simulink model "Fixed_Wing_Model"  (R2023a)
settings: Solver=FixedStepAuto  StartTime=0.0  StopTime=inf  FixedStep=model_sampling_time  RelTol=1e-3
InitFcn:
  | run("Parameters.m")
values from neighbouring files (symbols this model uses):
  Alpha = params.Aerodynamics.Alpha    [aircraft_model.m]    (also in aircraft_params.mat = [-0.698131700798 -0.680678408278 -0.663225115758 -0.64577182; cost_straight_level.m = atan2(X(3), X(1)); create_table.m = deg2rad(-40:1:40)'; nonlinear_const.m = atan2(X(3), X(1)))
  Beta = params.Aerodynamics.Beta    [aircraft_model.m]    (also in aircraft_params.mat = [-0.349065850399 -0.261799387799 -0.174532925199 -0.08726646; create_table.m = deg2rad(-20:5:20)')
  CD_alpha_beta = [0.0544509195029 0.0530405310175 0.0517292718774 0.0505171420827 0.0494041416333 0.0483902705292 0.0474755287703 0.0466599163568 0.0459434332887 0.0453260795658 0.0448078551882 0.0443887601559 ... (729 elements, 81x9)]    [aircraft_params.mat]    (also in create_table.m = zeros(length(Alpha), length(Beta)))
  CD_alpha_dot = 0    [Parameters.m]    (also in aircraft_params.mat)
  CD_u = 0    [Parameters.m]    (also in aircraft_params.mat)
  CDda = [0 0 0 0 0 0 0 0 0 0 0 0 ... (1539 elements, 19x81)]    [aircraft_params.mat]    (also in create_table.m = zeros(length(da), length(Alpha)))
  CDde = [0 0 0 0 0 0 0 0 0 0 0 0 ... (1539 elements, 19x81)]    [aircraft_params.mat]    (also in create_table.m = zeros(length(de), length(Alpha)))
  CDdr = [0 0 0 0 0 0 0 0 0 0 0 0 ... (171 elements, 19x9)]    [aircraft_params.mat]    (also in create_table.m = zeros(length(dr), length(Beta)))
  CDp = [0.00874 0.009614 0.010488 0.011362 0.012236 0.01311 0.013984 0.014858 0.015732 0.016606 0.01748 0.018354 ... (81 elements, 81x1)]    [aircraft_params.mat]    (also in create_table.m = zeros(length(Alpha),1))
  CDq = [0 0 0 0 0 0 0 0 0 0 0 0 ... (81 elements, 81x1)]    [aircraft_params.mat]    (also in create_table.m = zeros(length(Alpha),1))
  CDr = [0 0 0 0 0 0 0 0 0 0 0 0 ... (81 elements, 81x1)]    [aircraft_params.mat]    (also in create_table.m = zeros(length(Alpha),1))
  chord = 0.1894    [Parameters.m]    (also in aircraft_model.m = params.chord; aircraft_params.mat)
  CL_alpha_beta = [-0.633037607685 -0.615603980908 -0.597456739131 -0.578694538839 -0.559464427591 -0.54002303701 -0.520877191922 -0.503102694522 -0.489045924609 -0.483759795494 -0.497410215644 -0.54697394645 ... (729 elements, 81x9)]    [aircraft_params.mat]    (also in create_table.m = zeros(length(Alpha), length(Beta)))
  Cl_alpha_beta = [0.00837758040957 0.00921533845053 0.0100530964915 0.0108908545324 0.0117286125734 0.0125663706144 0.0134041286553 0.0142418866963 0.0150796447372 0.0159174027782 0.0167551608191 0.0175929188601 ... (729 elements, 81x9)]    [aircraft_params.mat]    (also in create_table.m = zeros(length(Alpha), length(Beta)))
  CL_alpha_dot = 0    [Parameters.m]    (also in aircraft_params.mat)
  Cl_alpha_dot = 0    [Parameters.m]    (also in aircraft_params.mat)
  CL_u = 0    [Parameters.m]    (also in aircraft_params.mat)
  Cl_u = 0    [Parameters.m]    (also in aircraft_params.mat)
  CLda = [0 0 0 0 0 0 0 0 0 0 0 0 ... (1539 elements, 19x81)]    [aircraft_params.mat]    (also in create_table.m = zeros(length(da), length(Alpha)))
  Clda = [-0.0125663706144 -0.0111701072128 -0.00977384381117 -0.00837758040957 -0.00698131700798 -0.00558505360638 -0.00418879020479 -0.00279252680319 -0.0013962634016 0 0.0013962634016 0.00279252680319 ... (1539 elements, 19x81)]    [aircraft_params.mat]    (also in create_table.m = zeros(length(da), length(Alpha)))
  CLde = [0.0565486677646 0.0502654824574 0.0439822971503 0.0376991118431 0.0314159265359 0.0251327412287 0.0188495559215 0.0125663706144 0.00628318530718 0 -0.00628318530718 -0.0125663706144 ... (1539 elements, 19x81)]    [aircraft_params.mat]    (also in create_table.m = zeros(length(de), length(Alpha)))
  Clde = [0 0 0 0 0 0 0 0 0 0 0 0 ... (1539 elements, 19x81)]    [aircraft_params.mat]    (also in create_table.m = zeros(length(de), length(Alpha)))
  CLdr = [0 0 0 0 0 0 0 0 0 0 0 0 ... (171 elements, 19x9)]    [aircraft_params.mat]    (also in create_table.m = zeros(length(dr), length(Beta)))
  Cldr = [-0.0758694625842 -0.0674395222971 -0.0590095820099 -0.0505796417228 -0.0421497014357 -0.0337197611485 -0.0252898208614 -0.0168598805743 -0.00842994028713 0 0.00842994028713 0.0168598805743 ... (171 elements, 19x9)]    [aircraft_params.mat]    (also in create_table.m = zeros(length(dr), length(Beta)))
  CLp = [0 0 0 0 0 0 0 0 0 0 0 0 ... (81 elements, 81x1)]    [aircraft_params.mat]    (also in create_table.m = zeros(length(Alpha),1))
  Clp = [-0.052 -0.0572 -0.0624 -0.0676 -0.0728 -0.078 -0.0832 -0.0884 -0.0936 -0.0988 -0.104 -0.1092 ... (81 elements, 81x1)]    [aircraft_params.mat]    (also in create_table.m = zeros(length(Alpha),1))
  CLq = [0 0 0 0 0 0 0 0 0 0 0 0 ... (81 elements, 81x1)]    [aircraft_params.mat]    (also in create_table.m = zeros(length(Alpha),1))
  Clq = [0 0 0 0 0 0 0 0 0 0 0 0 ... (81 elements, 81x1)]    [aircraft_params.mat]    (also in create_table.m = zeros(length(Alpha),1))
  CLr = [0 0 0 0 0 0 0 0 0 0 0 0 ... (81 elements, 81x1)]    [aircraft_params.mat]    (also in create_table.m = zeros(length(Alpha),1))
  Clr = [0.028 0.0308 0.0336 0.0364 0.0392 0.042 0.0448 0.0476 0.0504 0.0532 0.056 0.0588 ... (81 elements, 81x1)]    [aircraft_params.mat]    (also in create_table.m = zeros(length(Alpha),1))
  Cm_alpha_beta = [0.220686842599 0.214585171534 0.208483500469 0.202381829404 0.196280158339 0.190178487274 0.184076816209 0.177975145144 0.171873474079 0.165771803014 0.159670131949 0.153568460884 ... (729 elements, 81x9)]    [aircraft_params.mat]    (also in create_table.m = zeros(length(Alpha), length(Beta)))
  Cm_alpha_dot = 0    [Parameters.m]    (also in aircraft_params.mat)
  Cm_u = 0    [Parameters.m]    (also in aircraft_params.mat)
  Cmda = [0 0 0 0 0 0 0 0 0 0 0 0 ... (1539 elements, 19x81)]    [aircraft_params.mat]    (also in create_table.m = zeros(length(da), length(Alpha)))
  Cmde = [0.0785398163397 0.0698131700798 0.0610865238198 0.0523598775598 0.0436332312999 0.0349065850399 0.0261799387799 0.0174532925199 0.00872664625997 0 -0.00872664625997 -0.0174532925199 ... (1539 elements, 19x81)]    [aircraft_params.mat]    (also in create_table.m = zeros(length(de), length(Alpha)))
  Cmdr = [0 0 0 0 0 0 0 0 0 0 0 0 ... (171 elements, 19x9)]    [aircraft_params.mat]    (also in create_table.m = zeros(length(dr), length(Beta)))
  Cmp = [0 0 0 0 0 0 0 0 0 0 0 0 ... (81 elements, 81x1)]    [aircraft_params.mat]    (also in create_table.m = zeros(length(Alpha),1))
  Cmq = [-0.72 -0.792 -0.864 -0.936 -1.008 -1.08 -1.152 -1.224 -1.296 -1.368 -1.44 -1.512 ... (81 elements, 81x1)]    [aircraft_params.mat]    (also in create_table.m = zeros(length(Alpha),1))
  Cmr = [0 0 0 0 0 0 0 0 0 0 0 0 ... (81 elements, 81x1)]    [aircraft_params.mat]    (also in create_table.m = zeros(length(Alpha),1))
  Cn_alpha_beta = [-0.0174532925199 -0.0191986217719 -0.0209439510239 -0.0226892802759 -0.0244346095279 -0.0261799387799 -0.0279252680319 -0.0296705972839 -0.0314159265359 -0.0331612557879 -0.0349065850399 -0.0366519142919 ... (729 elements, 81x9)]    [aircraft_params.mat]    (also in create_table.m = zeros(length(Alpha), length(Beta)))
  Cn_alpha_dot = 0    [Parameters.m]    (also in aircraft_params.mat)
  Cn_u = 0    [Parameters.m]    (also in aircraft_params.mat)
  Cnda = [-0.00942477796077 -0.00837758040957 -0.00733038285838 -0.00628318530718 -0.00523598775598 -0.00418879020479 -0.00314159265359 -0.00209439510239 -0.0010471975512 0 0.0010471975512 0.00209439510239 ... (1539 elements, 19x81)]    [aircraft_params.mat]    (also in create_table.m = zeros(length(da), length(Alpha)))
  Cnde = [0 0 0 0 0 0 0 0 0 0 0 0 ... (1539 elements, 19x81)]    [aircraft_params.mat]    (also in create_table.m = zeros(length(de), length(Alpha)))
  Cndr = [0.0231221219304 0.0205529972715 0.0179838726125 0.0154147479536 0.0128456232947 0.0102764986357 0.00770737397681 0.00513824931787 0.00256912465894 0 -0.00256912465894 -0.00513824931787 ... (171 elements, 19x9)]    [aircraft_params.mat]    (also in create_table.m = zeros(length(dr), length(Beta)))
  Cnp = [0.0044 0.00484 0.00528 0.00572 0.00616 0.0066 0.00704 0.00748 0.00792 0.00836 0.0088 0.00924 ... (81 elements, 81x1)]    [aircraft_params.mat]    (also in create_table.m = zeros(length(Alpha),1))
  Cnq = [0 0 0 0 0 0 0 0 0 0 0 0 ... (81 elements, 81x1)]    [aircraft_params.mat]    (also in create_table.m = zeros(length(Alpha),1))
  Cnr = [-0.07 -0.077 -0.084 -0.091 -0.098 -0.105 -0.112 -0.119 -0.126 -0.133 -0.14 -0.147 ... (81 elements, 81x1)]    [aircraft_params.mat]    (also in create_table.m = zeros(length(Alpha),1))
  CY_alpha_beta = [0.0684169066782 0.075258597346 0.0821002880138 0.0889419786816 0.0957836693494 0.102625360017 0.109467050685 0.116308741353 0.123150432021 0.129992122689 0.136833813356 0.143675504024 ... (729 elements, 81x9)]    [aircraft_params.mat]    (also in create_table.m = zeros(length(Alpha), length(Beta)))
  CY_alpha_dot = 0    [Parameters.m]    (also in aircraft_params.mat)
  CY_u = 0    [Parameters.m]    (also in aircraft_params.mat)
  CYda = [0 0 0 0 0 0 0 0 0 0 0 0 ... (1539 elements, 19x81)]    [aircraft_params.mat]    (also in create_table.m = zeros(length(da), length(Alpha)))
  CYde = [0 0 0 0 0 0 0 0 0 0 0 0 ... (1539 elements, 19x81)]    [aircraft_params.mat]    (also in create_table.m = zeros(length(de), length(Alpha)))
  CYdr = [0.122836272755 0.109187798005 0.0955393232542 0.0818908485036 0.068242373753 0.0545938990024 0.0409454242518 0.0272969495012 0.0136484747506 0 -0.0136484747506 -0.0272969495012 ... (171 elements, 19x9)]    [aircraft_params.mat]    (also in create_table.m = zeros(length(dr), length(Beta)))
  CYp = [0 0 0 0 0 0 0 0 0 0 0 0 ... (81 elements, 81x1)]    [aircraft_params.mat]    (also in create_table.m = zeros(length(Alpha),1))
  CYq = [0 0 0 0 0 0 0 0 0 0 0 0 ... (81 elements, 81x1)]    [aircraft_params.mat]    (also in create_table.m = zeros(length(Alpha),1))
  CYr = [0 0 0 0 0 0 0 0 0 0 0 0 ... (81 elements, 81x1)]    [aircraft_params.mat]    (also in create_table.m = zeros(length(Alpha),1))
  D = zeros(size(B_long))    [Linearized_Model.m]    (also in linear_models.mat = [0 0 0 0 0 0 0 0 0 0 0 0 ... (16 elements, 4x4)])
  da = params.Aerodynamics.da    [aircraft_model.m]    (also in aircraft_params.mat = [-0.785398163397 -0.698131700798 -0.610865238198 -0.52359877; create_table.m = deg2rad(-45:5:45))
  da_lim = deg2rad(45)    [Parameters.m]    (also in aircraft_model.m = params.da_lim; aircraft_params.mat = 0.785398163397)
  de_lim = deg2rad(45)    [Parameters.m]    (also in aircraft_model.m = params.de_lim; aircraft_params.mat = 0.785398163397)
  dr = params.Aerodynamics.dr    [aircraft_model.m]    (also in aircraft_params.mat = [-0.785398163397 -0.698131700798 -0.610865238198 -0.52359877; create_table.m = deg2rad(-45:5:45))
  dr_lim = deg2rad(45)    [Parameters.m]    (also in aircraft_model.m = params.dr_lim; aircraft_params.mat = 0.785398163397)
  dth_lim = 100    [Parameters.m]    (also in aircraft_model.m = params.dth_lim; aircraft_params.mat)
  h_ref = 0    [Parameters.m]    (also in aircraft_params.mat)
  Inertia_Tensor = [Jx -Jxy -Jxz ... (first row only)    [Parameters.m]    (also in aircraft_model.m; aircraft_params.mat = [0.8244  0  -0.1204; 0  1.135  0; -0.1204  0  1.759])
  lat_ref_deg = 40    [Parameters.m]    (also in aircraft_params.mat)
  long_ref_deg = 20    [Parameters.m]    (also in aircraft_params.mat)
  mass = 13.5    [Parameters.m]    (also in aircraft_model.m = params.mass; aircraft_params.mat)
  Motor =     [aircraft_params.mat]
  pqr_initial = [0; 0; 0]    [Parameters.m]    (also in aircraft_params.mat = [0 0 0])
  quat_initial = eul2quat(euler_initial')    [Parameters.m]    (also in aircraft_params.mat = [1 0 0 0])
  rho_msl = 1.225    [Parameters.m]    (also in aircraft_model.m = params.rho_msl; aircraft_params.mat)
  S = 2.8956    [Parameters.m]    (also in aircraft_model.m = params.S; aircraft_params.mat)
  v_body_initial = [30; 0; 0]    [Parameters.m]    (also in aircraft_params.mat = [30 0 0])
  wing_span = 0.55    [Parameters.m]    (also in aircraft_model.m = params.wing_span; aircraft_params.mat)
undefined symbols (not defined in the file or in its folder): DiscIntNeverNeededParam, Earth, lat_deg, long_deg, WGS84
libraries: simulink x20, aerolibutil x5, matrix_library x2, aerolibtransform2 x2, sharedtransform x2, simulink_extras x2, sharedutil x1, aerolibatmos2 x1, aerolibsim3d x1, sim3dlib x1
(part 1 of 2)
settings Model: Creator=burak  LastModifiedBy=burak

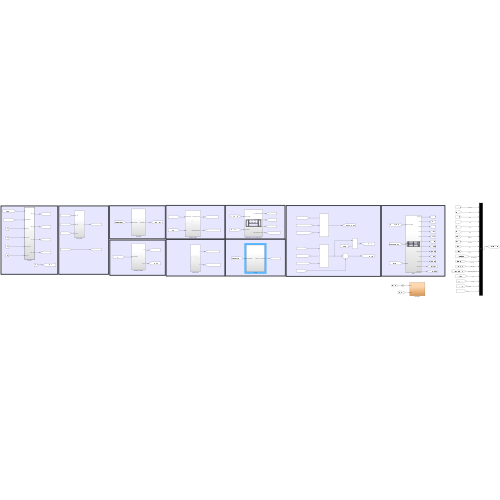
[thumbnail: Simulink's stored preview of the top-level diagram]
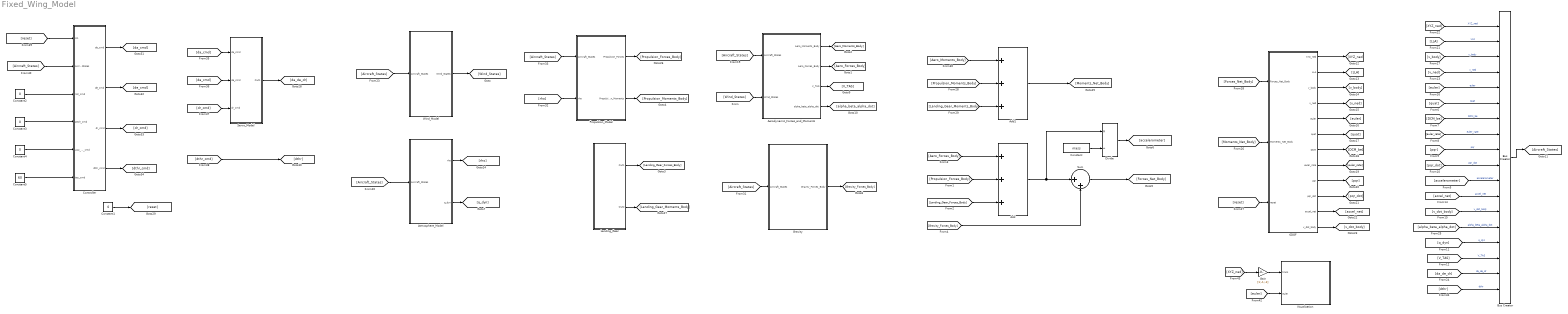
== system Fixed_Wing_Model ==
  6DOF : Subsystem
  Add : Sum  Inputs=+++
  Add1 : Sum  Inputs=+++
  Aerodynamic_Forces_and_Moments : Subsystem
  Atmosphere_Model : Subsystem
  Bus Creator : BusCreator  Inputs=18
  Constant : Constant  Value=mass
  Constant{1..4} (4 alike) : Constant  Value=0
  Constant5 : Constant  Value=60
  Controller : Subsystem  TreatAsAtomicUnit=on  SystemSampleTime=1/50
  Divide : Product  Inputs=*/
  Gain : Gain  Gain=[1;-1;-1]
  Gravity : Subsystem
  Landing_Gear : Subsystem
  Propulsion_Model : Subsystem
  Servo_Model : Subsystem
  Sum : Sum  Inputs=|++
  Visualization : Subsystem
  Wind_Model : Subsystem
  wires:
  Wind_Model/1(Wind_States) -> [Wind_States]
  [Wind_States] -> Aerodynamic_Forces_and_Moments/2(Wind_States)
  6DOF/1(XYZ_ned) -> [XYZ_ned]
  6DOF/2(LLA) -> [LLA]
  6DOF/12(v_dot_body) -> [v_dot_body]
  6DOF/11(accel_net) -> [accel_net]
  6DOF/10(pqr_dot) -> [pqr_dot]
  6DOF/9(pqr) -> [pqr]
  6DOF/8(euler_rate) -> [euler_rate]
  6DOF/7(DCM) -> [DCM_be]
  6DOF/6(quat) -> [quat]
  6DOF/5(euler) -> [euler]
  6DOF/4(v_ned) -> [v_ned]
  6DOF/3(v_body) -> [v_body]
  Gravity/1(Gravity_Forces_Body) -> [Gravity_Forces_Body]
  Aerodynamic_Forces_and_Moments/2(Aero_Forces_Body) -> [Aero_Forces_Body]
  Aerodynamic_Forces_and_Moments/1(Aero_Moments_Body) -> [Aero_Moments_Body]
  Landing_Gear/1(Out1) -> [Landing_Gear_Forces_Body]
  Propulsion_Model/2(Propulsion_Moments) -> [Propulsion_Moments_Body]
  [Aero_Forces_Body] -> Add/1
  [Propulsion_Forces_Body] -> Add/2
  [Landing_Gear_Forces_Body] -> Add/3
  Add/1 -> Divide/1, Sum/1
  [Gravity_Forces_Body] -> Sum/2
  Sum/1 -> [Forces_Net_Body]
  Divide/1 -> [accelerometer]
  Atmosphere_Model/2(q_dyn) -> [q_dyn]
  Aerodynamic_Forces_and_Moments/3(V_TAS) -> [V_TAS]
  Aerodynamic_Forces_and_Moments/4(alpha_beta_alpha_dot) -> [alpha_beta_alpha_dot]
  [XYZ_ned] -> Bus Creator/1  "XYZ_ned"
  [V_TAS] -> Bus Creator/16  "V_TAS"
  [LLA] -> Bus Creator/2  "LLA"
  [v_body] -> Bus Creator/3  "v_body"
  [v_ned] -> Bus Creator/4  "v_ned"
  [euler] -> Bus Creator/5  "euler"
  [quat] -> Bus Creator/6  "quat"
  [DCM_be] -> Bus Creator/7  "DCM_be"
  [euler_rate] -> Bus Creator/8  "euler_rate"
  [pqr] -> Bus Creator/9  "pqr"
  [pqr_dot] -> Bus Creator/10  "pqr_dot"
  [accelerometer] -> Bus Creator/11  "accelerometer"
  [accel_net] -> Bus Creator/12  "accel_net"
  [v_dot_body] -> Bus Creator/13  "v_dot_body"
  [alpha_beta_alpha_dot] -> Bus Creator/14  "alpha_beta_alpha_dot"
  [q_dyn] -> Bus Creator/15  "q_dyn"
  [Aircraft_States] -> Aerodynamic_Forces_and_Moments/1(Aircraft_States)
  Bus Creator/1 -> [Aircraft_States]
  [Aircraft_States] -> Atmosphere_Model/1(Aircraft_States)
  Atmosphere_Model/1(rho) -> [rho]
  [Aircraft_States] -> Wind_Model/1(Aircraft_States)
  [da_de_dr] -> Bus Creator/17  "da_de_dr"
  Constant/1 -> Divide/2
  [Forces_Net_Body] -> 6DOF/1(Forces_Net_Body)
  [Moments_Net_Body] -> 6DOF/2(Moments_Net_Body)
  [reset] -> 6DOF/3(reset)
  Add1/1 -> [Moments_Net_Body]
  [Propulsion_Moments_Body] -> Add1/2
  [Aero_Moments_Body] -> Add1/1
  [Landing_Gear_Moments_Body] -> Add1/3
  [Aircraft_States] -> Gravity/1(Aircraft_States)
  Propulsion_Model/1(Propulsion_Forces) -> [Propulsion_Forces_Body]
  Landing_Gear/2(Out2) -> [Landing_Gear_Moments_Body]
  Servo_Model/1(Out1) -> [da_de_dr]
  Constant1/1 -> [reset]
  [rho] -> Propulsion_Model/2(rho)
  [Aircraft_States] -> Propulsion_Model/1(Aircraft_States)
  [dthr] -> Bus Creator/18  "dthr"
  Controller/1(da_cmd) -> [da_cmd]
  Controller/2(de_cmd) -> [de_cmd]
  Controller/3(dr_cmd) -> [dr_cmd]
  Controller/4(dthr_cmd) -> [dthr_cmd]
  [reset] -> Controller/1(In1)
  [Aircraft_States] -> Controller/2(Aircraft_States)
  [XYZ_ned] -> Gain/1
  [euler] -> Visualization/2(euler)
  Gain/1 -> Visualization/1(trans)
  Constant5/1 -> Controller/6(tas_cmd)
  Constant4/1 -> Controller/5(yaw_rate_cmd)
  Constant3/1 -> Controller/4(pitch_cmd)
  Constant2/1 -> Controller/3(roll_cmd)
  [de_cmd] -> Servo_Model/2(de_cmd)
  [dr_cmd] -> Servo_Model/3(dr_cmd)
  [dthr_cmd] -> [dthr]
  [da_cmd] -> Servo_Model/1(da_cmd)

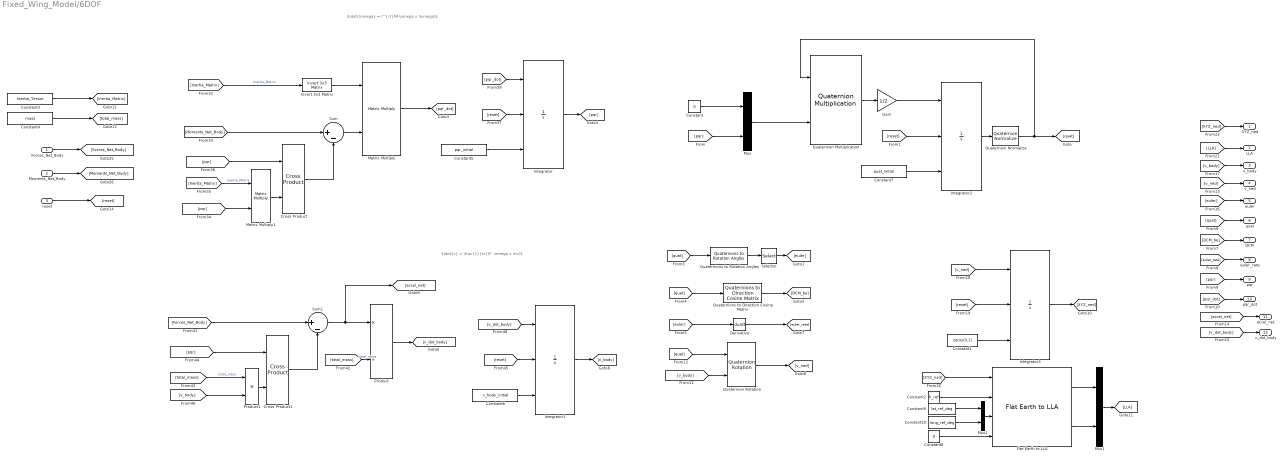
== system Fixed_Wing_Model/6DOF ==
  note: $\dot{v} = \frac{1}{m}(F- \omega x mv)$
  note: $\dot{\omega} = I^{-1}(M-\omega x I\omega)$
  Forces_Net_Body : Inport
  Moments_Net_Body : Inport  Port=2
  reset : Inport  Port=3
  Constant : Constant  Value=0
  Constant1 : Constant  Value=zeros(3,1)
  Constant10 : Constant  Value=long_ref_deg
  Constant2 : Constant  Value=h_ref
  Constant3 : Constant  Value=Inertia_Tensor
  Constant4 : Constant  Value=mass
  Constant5 : Constant  Value=pqr_initial
  Constant6 : Constant  Value=v_body_initial
  Constant7 : Constant  Value=quat_initial
  Constant8 : Constant  Value=0
  Constant9 : Constant  Value=lat_ref_deg
  Cross Product : matrix_library/Cross Product
  Cross Product1 : matrix_library/Cross Product
  Derivative : Derivative
  Flat Earth to LLA : aerolibtransform2/Flat Earth to LLA  units=Metric (MKS)  ptype=Earth (WGS84)  F=1/298.257223563  R=6378137  refPosPort=on  LL0=[lat_deg long_deg]  psi=0
  Gain : Gain  Gain=1/2
  Integrator{,1..3} (4 alike) : Integrator  ExternalReset=rising  InitialConditionSource=external
  Invert 3x3 Matrix : aerolibutil/Invert  3x3 Matrix
  Matrix Multiply : Product  Multiplication=Matrix(*)
  Matrix Multiply1 : Product  Multiplication=Matrix(*)
  Mux : Mux  Inputs=2
  Mux1 : Mux  Inputs=2
  Mux2 : Mux  Inputs=2
  Product : Product  Inputs=*/
  Product1 : Product
  Quaternion Multiplication : aerolibutil/Quaternion Multiplication
  Quaternion Normalize : sharedutil/Quaternion Normalize  aMode=aMode
  Quaternion Rotation : aerolibutil/Quaternion Rotation
  Quaternions to Direction Cosine Matrix : sharedtransform/Quaternions to  Direction Cosine Matrix  aMode=aMode
      settings: LibrarySourceBlock=|
      | aerolibtransform2/Quaternions to
      | Direction Cosine Matrix
  Quaternions to Rotation Angles : sharedtransform/Quaternions to Rotation Angles  rotationOrder=ZYX  aMode=aMode
  Selector : Selector  InputPortWidth=3  IndexOptions=Index vector (dialog)  Indices=[3 2 1]  OutputSizes=1
  Sum : Sum  Inputs=|+-
  Sum1 : Sum  Inputs=|+-
  XYZ_ned : Outport
  LLA : Outport  Port=2
  v_body : Outport  Port=3
  v_ned : Outport  Port=4
  euler : Outport  Port=5
  quat : Outport  Port=6
  DCM : Outport  Port=7
  euler_rate : Outport  Port=8
  pqr : Outport  Port=9
  pqr_dot : Outport  Port=10
  accel_net : Outport  Port=11
  v_dot_body : Outport  Port=12
  wires:
  Mux/1 -> Quaternion Multiplication/2
  Derivative/1 -> [euler_rate]
  [euler] -> Derivative/1
  Integrator1/1 -> [v_body]
  Quaternion Normalize/1 -> Quaternion Multiplication/1, [quat]
  Gain/1 -> Integrator2/1
  Integrator/1 -> [pqr]
  Integrator2/1 -> Quaternion Normalize/1
  [pqr_dot] -> Integrator/1
  Quaternions to Rotation Angles/1 -> Selector/1
  [Inertia_Matrix] -> Matrix Multiply1/1  "Inertia_Matrix"
  Invert 3x3 Matrix/1 -> Matrix Multiply/1
  [pqr] -> Mux/2
  [Inertia_Matrix] -> Invert 3x3 Matrix/1  "Inertia_Matrix"
  [quat] -> Quaternions to Direction Cosine Matrix/1
  [quat] -> Quaternions to Rotation Angles/1
  [total_mass] -> Product1/1  "total_mass"
  Matrix Multiply/1 -> [pqr_dot]
  Constant/1 -> Mux/1
  Matrix Multiply1/1 -> Cross Product/2
  Selector/1 -> [euler]
  [reset] -> Integrator/2
  Sum/1 -> Matrix Multiply/2
  [total_mass] -> Product/2  "total_mass"
  [reset] -> Integrator1/2
  Quaternion Multiplication/1 -> Gain/1
  Constant7/1 -> Integrator2/3
  Constant5/1 -> Integrator/3
  Cross Product1/1 -> Sum1/2
  [pqr] -> Matrix Multiply1/2
  Quaternions to Direction Cosine Matrix/1 -> [DCM_be]
  Cross Product/1 -> Sum/2
  [Moments_Net_Body] -> Sum/1
  [pqr] -> Cross Product1/1
  Sum1/1 -> [accel_net], Product/1
  [Forces_Net_Body] -> Sum1/1
  Product1/1 -> Cross Product1/2
  [v_body] -> Product1/2
  Constant6/1 -> Integrator1/3
  [reset] -> Integrator2/2
  Product/1 -> [v_dot_body]
  [v_dot_body] -> Integrator1/1
  [pqr] -> Cross Product/1
  [v_body] -> Quaternion Rotation/2
  [quat] -> Quaternion Rotation/1
  Quaternion Rotation/1 -> [v_ned]
  [v_ned] -> Integrator3/1
  [reset] -> Integrator3/2
  Constant1/1 -> Integrator3/3
  Integrator3/1 -> [XYZ_ned]
  [XYZ_ned] -> Flat Earth to LLA/1
  Constant2/1 -> Flat Earth to LLA/2
  [XYZ_ned] -> XYZ_ned/1
  [LLA] -> LLA/1
  [v_body] -> v_body/1
  [v_ned] -> v_ned/1
  [euler] -> euler/1
  [quat] -> quat/1
  [DCM_be] -> DCM/1
  [euler_rate] -> euler_rate/1
  [pqr] -> pqr/1
  [pqr_dot] -> pqr_dot/1
  [accel_net] -> accel_net/1
  [v_dot_body] -> v_dot_body/1
  Forces_Net_Body/1 -> [Forces_Net_Body]
  Moments_Net_Body/1 -> [Moments_Net_Body]
  Constant3/1 -> [Inertia_Matrix]
  Constant4/1 -> [total_mass]
  reset/1 -> [reset]
  Constant8/1 -> Flat Earth to LLA/4
  Mux2/1 -> Flat Earth to LLA/3
  Constant9/1 -> Mux2/1
  Constant10/1 -> Mux2/2
  Flat Earth to LLA/1 -> Mux1/1
  Flat Earth to LLA/2 -> Mux1/2
  Mux1/1 -> [LLA]

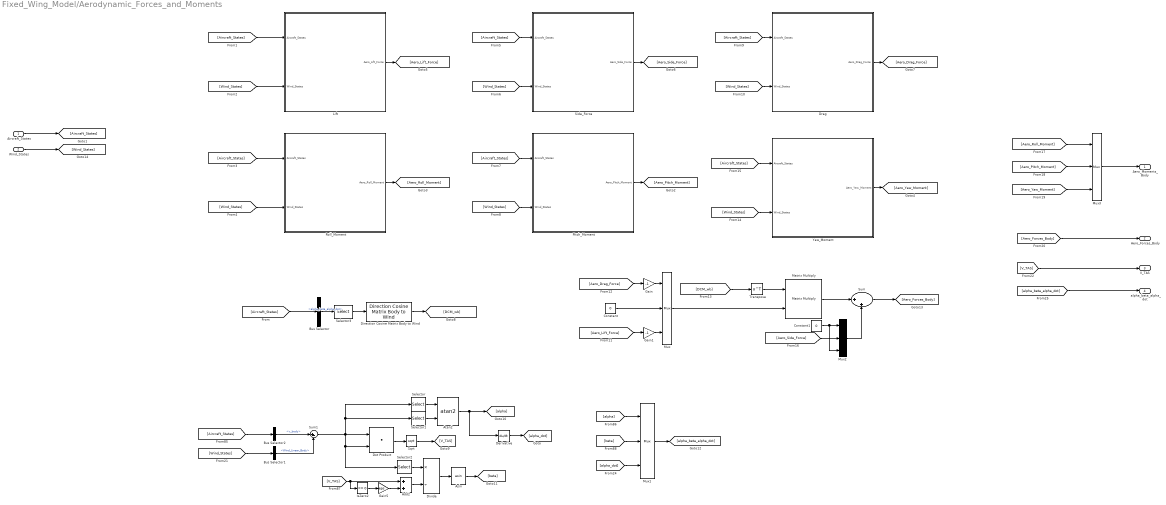
== system Fixed_Wing_Model/Aerodynamic_Forces_and_Moments ==
  Aircraft_States : Inport
  Wind_States : Inport  Port=2
  Add2 : Sum
  Asin : Trigonometry  Operator=asin
  Atan2 : Trigonometry  Operator=atan2
  Bus Selector : BusSelector  OutputSignals=alpha_beta_alpha_dot
  Bus Selector1 : BusSelector  OutputSignals=Wind_Linear_Body
  Bus Selector2 : BusSelector  OutputSignals=v_body
  Constant : Constant  Value=0
  Constant1 : Constant  Value=0
  Derivative : Derivative
  Direction Cosine Matrix Body to Wind : aerolibtransform2/Direction Cosine Matrix Body to Wind
  Divide : Product  Inputs=*/
  Dot Product : DotProduct  OutDataTypeStr=Inherit: Inherit via internal rule
  Drag : Subsystem
  Gain : Gain  Gain=-1
  Gain1 : Gain  Gain=-1
  Gain5 : Gain  Gain=eps
  IsZero2 : simulink/Logic and Bit Operations/Compare To Zero  relop===  OutDataTypeStr=uint8
      settings: LibrarySourceBlock=|
      | simulink/Quick Insert/Logic and Bit
      | Operations/IsZero
  Lift : Subsystem
  Matrix Multiply : Product  Multiplication=Matrix(*)
  Mux{,1..3} (4 alike) : Mux  Inputs=3
  Pitch_Moment : Subsystem
  Roll_Moment : Subsystem
  Selector : Selector  InputPortWidth=3  IndexOptions=Index vector (dialog)  Indices=3  OutputSizes=1
  Selector1 : Selector  InputPortWidth=3  IndexOptions=Index vector (dialog)  Indices=1  OutputSizes=1
  Selector2 : Selector  InputPortWidth=3  IndexOptions=Index vector (dialog)  Indices=2  OutputSizes=1
  Selector3 : Selector  InputPortWidth=3  IndexOptions=Index vector (dialog)  Indices=[1 2]  OutputSizes=1
  Side_Force : Subsystem
  Sqrt : Sqrt
  Sum : Sum  Inputs=|++
  Sum1 : Sum  Inputs=|+-
  Transpose : Math  Operator=transpose
  Yaw_Moment : Subsystem
  Aero_Moments_Body : Outport
  Aero_Forces_Body : Outport  Port=2
  V_TAS : Outport  Port=3
  alpha_beta_alpha_dot : Outport  Port=4
  wires:
  Atan2/1 -> [alpha], Derivative/1
  Gain5/1 -> Add2/2
  Dot Product/1 -> Sqrt/1
  IsZero2/1 -> Gain5/1
  Asin/1 -> [beta]
  Divide/1 -> Asin/1
  Add2/1 -> Divide/2
  [V_TAS] -> Add2/1, IsZero2/1
  Selector1/1 -> Atan2/2
  Selector/1 -> Atan2/1
  Sqrt/1 -> [V_TAS]
  Selector2/1 -> Divide/1
  [alpha] -> Mux1/1
  Mux1/1 -> [alpha_beta_alpha_dot]
  [beta] -> Mux1/2
  [Aero_Drag_Force] -> Gain/1
  [Aero_Pitch_Moment] -> Mux3/2
  Gain1/1 -> Mux/3
  Sum/1 -> [Aero_Forces_Body]
  [Aero_Side_Force] -> Mux2/2
  Gain/1 -> Mux/1
  Constant/1 -> Mux/2
  Matrix Multiply/1 -> Sum/1
  Transpose/1 -> Matrix Multiply/1
  [Aero_Forces_Body] -> Aero_Forces_Body/1
  Mux2/1 -> Sum/2
  [Aero_Yaw_Moment] -> Mux3/3
  Mux/1 -> Matrix Multiply/2
  Mux3/1 -> Aero_Moments_Body/1
  Constant1/1 -> Mux2/3, Mux2/1
  [Aero_Lift_Force] -> Gain1/1
  [DCM_wb] -> Transpose/1
  Bus Selector/1 -> Selector3/1  "<alpha_beta_alpha_dot>"
  [Aero_Roll_Moment] -> Mux3/1
  [Aircraft_States] -> Bus Selector/1
  Direction Cosine Matrix Body to Wind/1 -> [DCM_wb]
  Selector3/1 -> Direction Cosine Matrix Body to Wind/1
  Roll_Moment/1(Aero_Roll_Moment) -> [Aero_Roll_Moment]
  Aircraft_States/1 -> [Aircraft_States]
  Pitch_Moment/1(Aero_Pitch_Moment) -> [Aero_Pitch_Moment]
  Yaw_Moment/1(Aero_Yaw_Moment) -> [Aero_Yaw_Moment]
  Lift/1(Aero_Lift_Force) -> [Aero_Lift_Force]
  Side_Force/1(Aero_Side_Force) -> [Aero_Side_Force]
  Drag/1(Aero_Drag_Force) -> [Aero_Drag_Force]
  Wind_States/1 -> [Wind_States]
  [Aircraft_States] -> Lift/1(Aircraft_States)
  [Wind_States] -> Lift/2(Wind_States)
  [Aircraft_States] -> Roll_Moment/1(Aircraft_States)
  [Wind_States] -> Roll_Moment/2(Wind_States)
  [Aircraft_States] -> Side_Force/1(Aircraft_States)
  [Wind_States] -> Side_Force/2(Wind_States)
  [Aircraft_States] -> Pitch_Moment/1(Aircraft_States)
  [Wind_States] -> Pitch_Moment/2(Wind_States)
  [Aircraft_States] -> Drag/1(Aircraft_States)
  [Wind_States] -> Drag/2(Wind_States)
  [Aircraft_States] -> Yaw_Moment/1(Aircraft_States)
  [Wind_States] -> Yaw_Moment/2(Wind_States)
  [V_TAS] -> V_TAS/1
  [alpha_beta_alpha_dot] -> alpha_beta_alpha_dot/1
  [Aircraft_States] -> Bus Selector2/1
  [Wind_States] -> Bus Selector1/1
  Bus Selector2/1 -> Sum1/1  "<v_body>"
  Bus Selector1/1 -> Sum1/2  "<Wind_Linear_Body>"
  Sum1/1 -> Selector1/1, Selector/1, Selector2/1, Dot Product/2, Dot Product/1
  [alpha_dot] -> Mux1/3
  Derivative/1 -> [alpha_dot]

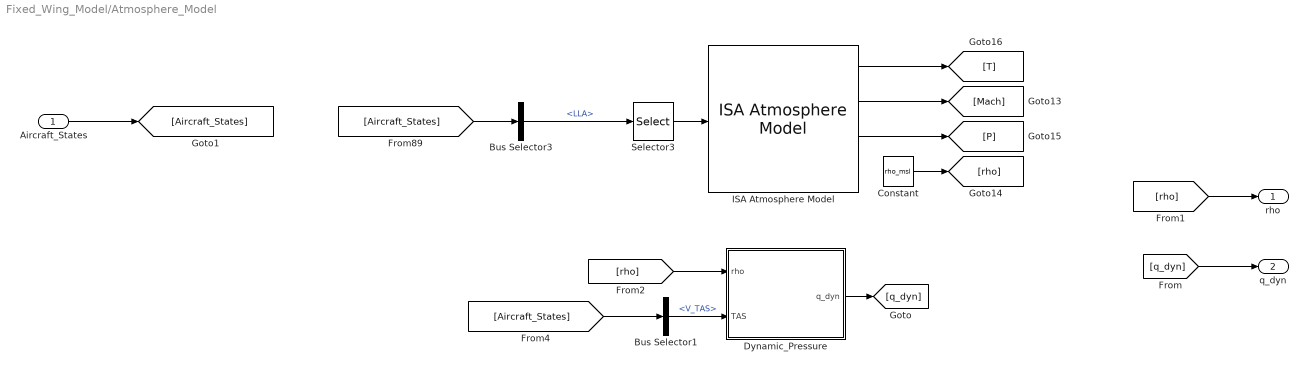
== system Fixed_Wing_Model/Atmosphere_Model ==
  Aircraft_States : Inport
  Bus Selector1 : BusSelector  OutputSignals=V_TAS
  Bus Selector3 : BusSelector  OutputSignals=LLA
  Constant : Constant  Value=rho_msl
  Dynamic_Pressure : Subsystem
  ISA Atmosphere Model : aerolibatmos2/ISA Atmosphere Model  custom=off  g=9.80665  gamma=1.4  R=287.0531  L=0.0065  h_trop=11000  h_strat=20000  rho0=1.225  P0=101325  T0=288.15  h0=0
  Selector3 : Selector  InputPortWidth=3  IndexOptions=Index vector (dialog)  Indices=3  OutputSizes=1
  rho : Outport
  q_dyn : Outport  Port=2
  wires:
  [Aircraft_States] -> Bus Selector3/1
  ISA Atmosphere Model/3 -> [P]
  Selector3/1 -> ISA Atmosphere Model/1
  ISA Atmosphere Model/2 -> [Mach]
  Bus Selector3/1 -> Selector3/1  "<LLA>"
  ISA Atmosphere Model/1 -> [T]
  [rho] -> Dynamic_Pressure/1(rho)
  Dynamic_Pressure/1(q_dyn) -> [q_dyn]
  [rho] -> rho/1
  [q_dyn] -> q_dyn/1
  Aircraft_States/1 -> [Aircraft_States]
  [Aircraft_States] -> Bus Selector1/1
  Bus Selector1/1 -> Dynamic_Pressure/2(TAS)  "<V_TAS>"
  Constant/1 -> [rho]

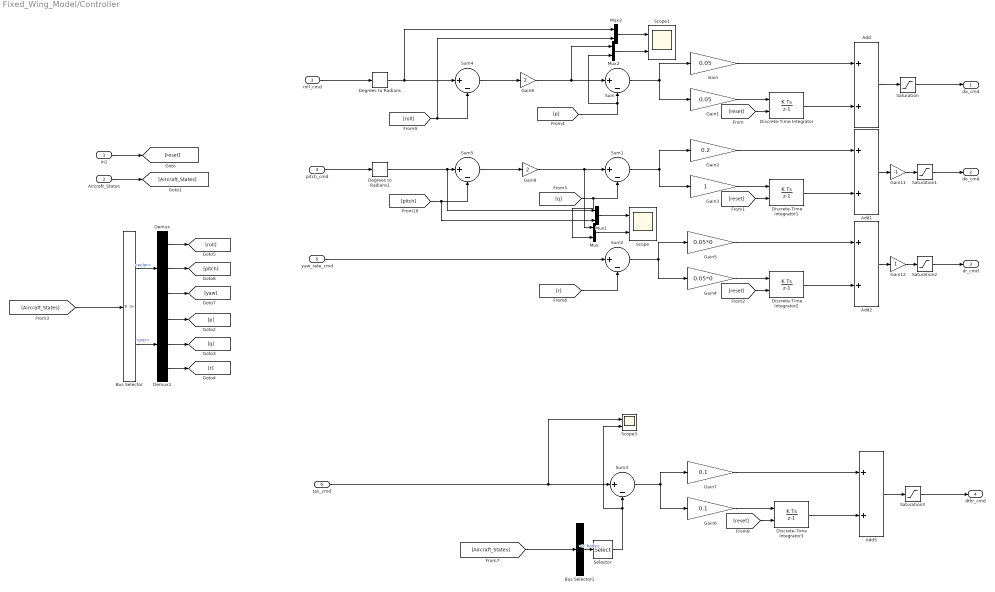
== system Fixed_Wing_Model/Controller ==
  In1 : Inport
  Aircraft_States : Inport  Port=2
  roll_cmd : Inport  Port=3
  pitch_cmd : Inport  Port=4
  yaw_rate_cmd : Inport  Port=5
  tas_cmd : Inport  Port=6
  Add{,1..3} (4 alike) : Sum
  Bus Selector : BusSelector  OutputSignals=euler,pqr
  Bus Selector1 : BusSelector  OutputSignals=v_body
  Degrees to Radians : simulink_extras/Transformations/Degrees to Radians
  Degrees to Radians1 : simulink_extras/Transformations/Degrees to Radians
  Demux : Demux  Outputs=3
  Demux1 : Demux  Outputs=3
  Discrete-Time Integrator : DiscreteIntegrator  ExternalReset=rising  SampleTime=-1  LimitOutput=on  UpperSaturationLimit=da_lim  LowerSaturationLimit=-da_lim  ICPrevOutput=DiscIntNeverNeededParam  ICPrevScaledInput=DiscIntNeverNeededParam
  Discrete-Time Integrator1 : DiscreteIntegrator  ExternalReset=rising  SampleTime=-1  LimitOutput=on  UpperSaturationLimit=de_lim  LowerSaturationLimit=-de_lim  ICPrevOutput=DiscIntNeverNeededParam  ICPrevScaledInput=DiscIntNeverNeededParam
  Discrete-Time Integrator2 : DiscreteIntegrator  ExternalReset=rising  SampleTime=-1  LimitOutput=on  UpperSaturationLimit=dr_lim  LowerSaturationLimit=-dr_lim  ICPrevOutput=DiscIntNeverNeededParam  ICPrevScaledInput=DiscIntNeverNeededParam
  Discrete-Time Integrator3 : DiscreteIntegrator  ExternalReset=rising  SampleTime=-1  LimitOutput=on  UpperSaturationLimit=dth_lim  LowerSaturationLimit=0  ICPrevOutput=DiscIntNeverNeededParam  ICPrevScaledInput=DiscIntNeverNeededParam
  Gain : Gain  Gain=0.05
  Gain1 : Gain  Gain=0.05
  Gain11 : Gain  Gain=-1
  Gain12 : Gain
  Gain2 : Gain  Gain=0.2
  Gain3 : Gain
  Gain4 : Gain  Gain=0.05*0
  Gain5 : Gain  Gain=0.05*0
  Gain6 : Gain  Gain=0.1
  Gain7 : Gain  Gain=0.1
  Gain8 : Gain  Gain=2
  Gain9 : Gain  Gain=2
  Mux{,1..3} (4 alike) : Mux  Inputs=2
  Saturation : Saturate  UpperLimit=da_lim  LowerLimit=-da_lim
  Saturation1 : Saturate  UpperLimit=de_lim  LowerLimit=-de_lim
  Saturation2 : Saturate  UpperLimit=dr_lim  LowerLimit=-dr_lim
  Saturation3 : Saturate  UpperLimit=dth_lim  LowerLimit=0
  Scope : Scope  NumInputPorts=2
  Scope1 : Scope  NumInputPorts=2
  Scope3 : Scope  NumInputPorts=2
  Selector : Selector  InputPortWidth=3  IndexOptions=Index vector (dialog)  Indices=1  OutputSizes=1
  Sum{,1..5} (6 alike) : Sum  Inputs=|+-
  da_cmd : Outport
  de_cmd : Outport  Port=2
  dr_cmd : Outport  Port=3
  dthr_cmd : Outport  Port=4
  wires:
  Add/1 -> Saturation/1
  Saturation1/1 -> de_cmd/1
  Saturation2/1 -> dr_cmd/1
  Saturation3/1 -> dthr_cmd/1
  Discrete-Time Integrator/1 -> Add/2
  Saturation/1 -> da_cmd/1
  Discrete-Time Integrator1/1 -> Add1/2
  Add1/1 -> Gain11/1
  Add2/1 -> Gain12/1
  Discrete-Time Integrator2/1 -> Add2/2
  Discrete-Time Integrator3/1 -> Add3/2
  Add3/1 -> Saturation3/1
  Gain/1 -> Add/1
  Gain1/1 -> Discrete-Time Integrator/1
  Gain2/1 -> Add1/1
  Gain3/1 -> Discrete-Time Integrator1/1
  Gain4/1 -> Discrete-Time Integrator2/1
  Gain5/1 -> Add2/1
  Gain6/1 -> Discrete-Time Integrator3/1
  In1/1 -> [reset]
  [reset] -> Discrete-Time Integrator/2
  [reset] -> Discrete-Time Integrator1/2
  [reset] -> Discrete-Time Integrator2/2
  Sum/1 -> Gain/1, Gain1/1
  Sum1/1 -> Gain2/1, Gain3/1
  Sum2/1 -> Gain5/1, Gain4/1
  Gain7/1 -> Add3/1
  Sum3/1 -> Gain7/1, Gain6/1
  Aircraft_States/1 -> [Aircraft_States]
  [Aircraft_States] -> Bus Selector/1
  Bus Selector/1 -> Demux/1  "<euler>"
  Bus Selector/2 -> Demux1/1  "<pqr>"
  Demux1/1 -> [p]
  Demux1/2 -> [q]
  Demux1/3 -> [r]
  Demux/1 -> [roll]
  Demux/2 -> [pitch]
  Demux/3 -> [yaw]
  [q] -> Mux/2, Sum1/2
  [r] -> Sum2/2
  [Aircraft_States] -> Bus Selector1/1
  Bus Selector1/1 -> Selector/1  "<v_body>"
  [reset] -> Discrete-Time Integrator3/2
  Sum4/1 -> Gain8/1
  Gain8/1 -> Mux2/1, Sum/1
  Sum5/1 -> Gain9/1
  [roll] -> Mux3/2, Sum4/2
  [pitch] -> Mux1/2, Sum5/2
  roll_cmd/1 -> Degrees to Radians/1
  Degrees to Radians/1 -> Mux3/1, Sum4/1
  Degrees to Radians1/1 -> Mux1/1, Sum5/1
  pitch_cmd/1 -> Degrees to Radians1/1
  tas_cmd/1 -> Scope3/1, Sum3/1
  Mux/1 -> Scope/2
  Mux1/1 -> Scope/1
  Gain11/1 -> Saturation1/1
  Gain9/1 -> Mux/1, Sum1/1
  Mux3/1 -> Scope1/1
  Mux2/1 -> Scope1/2
  [p] -> Sum/2, Mux2/2
  Gain12/1 -> Saturation2/1
  Selector/1 -> Scope3/2, Sum3/2
  yaw_rate_cmd/1 -> Sum2/1

== system Fixed_Wing_Model/Gravity ==
  Aircraft_States : Inport
  Bus Selector1 : BusSelector  OutputSignals=quat
  Constant : Constant  Value=[0;0;9.81]
  Gain : Gain  Gain=mass
  Quaternion Rotation : aerolibutil/Quaternion Rotation
  Gravity_Forces_Body : Outport
  wires:
  [Aircraft_States] -> Bus Selector1/1
  Bus Selector1/1 -> Quaternion Rotation/1  "<quat>"
  Quaternion Rotation/1 -> Gravity_Forces_Body/1
  Aircraft_States/1 -> [Aircraft_States]
  Constant/1 -> Gain/1
  Gain/1 -> Quaternion Rotation/2

== system Fixed_Wing_Model/Landing_Gear ==
  Constant1 : Constant  Value=zeros(3,1)
  Constant2 : Constant  Value=zeros(3,1)
  Out1 : Outport
  Out2 : Outport  Port=2
  wires:
  Constant1/1 -> Out1/1
  Constant2/1 -> Out2/1

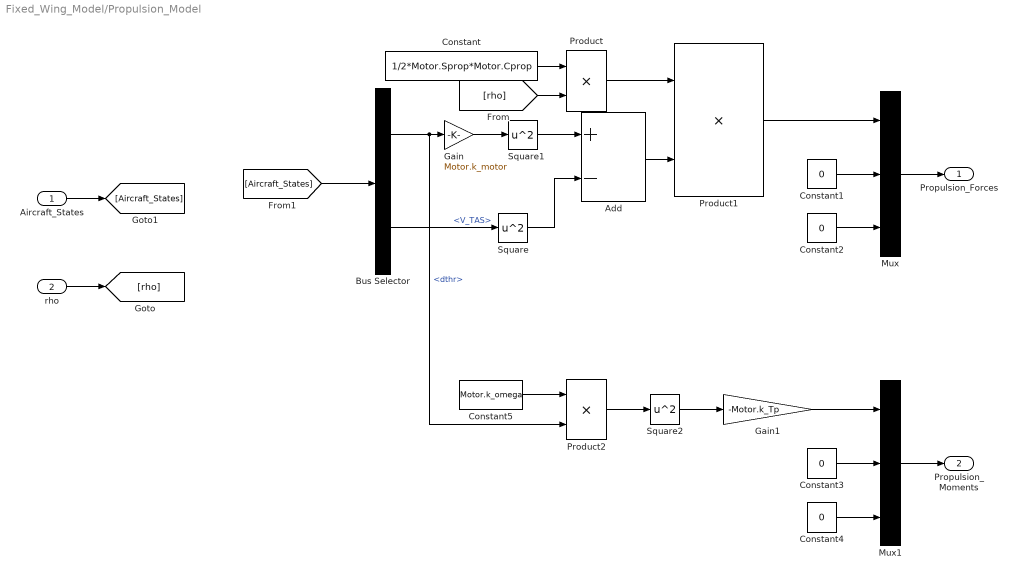
== system Fixed_Wing_Model/Propulsion_Model ==
  Aircraft_States : Inport
  rho : Inport  Port=2
  Add : Sum  Inputs=+-
  Bus Selector : BusSelector  OutputSignals=dthr,V_TAS
  Constant : Constant  Value=1/2*Motor.Sprop*Motor.Cprop
  Constant{1..4} (4 alike) : Constant  Value=0
  Constant5 : Constant  Value=Motor.k_omega
  Gain : Gain  Gain=Motor.k_motor
  Gain1 : Gain  Gain=-Motor.k_Tp
  Mux : Mux  Inputs=3
  Mux1 : Mux  Inputs=3
  Product : Product
  Product1 : Product
  Product2 : Product
  Square : Math  Operator=square
  Square1 : Math  Operator=square
  Square2 : Math  Operator=square
  Propulsion_Forces : Outport
  Propulsion_Moments : Outport  Port=2
  wires:
  Mux/1 -> Propulsion_Forces/1
  Constant/1 -> Product/1
  rho/1 -> [rho]
  [rho] -> Product/2
  Product/1 -> Product1/1
  Add/1 -> Product1/2
  Aircraft_States/1 -> [Aircraft_States]
  [Aircraft_States] -> Bus Selector/1
  Bus Selector/2 -> Square/1  "<V_TAS>"
  Square/1 -> Add/2
  Bus Selector/1 -> Product2/2, Gain/1  "<dthr>"
  Square1/1 -> Add/1
  Gain/1 -> Square1/1
  Product1/1 -> Mux/1
  Constant1/1 -> Mux/2
  Constant2/1 -> Mux/3
  Constant4/1 -> Mux1/3
  Constant3/1 -> Mux1/2
  Gain1/1 -> Mux1/1
  Mux1/1 -> Propulsion_Moments/1
  Product2/1 -> Square2/1
  Square2/1 -> Gain1/1
  Constant5/1 -> Product2/1

== system Fixed_Wing_Model/Servo_Model ==
  da_cmd : Inport
  de_cmd : Inport  Port=2
  dr_cmd : Inport  Port=3
  Mux : Mux  Inputs=3
  Transfer Fcn : TransferFcn  Numerator=[10]  Denominator=[1 10]
  Transfer Fcn1 : TransferFcn  Numerator=[10]  Denominator=[1 10]
  Transfer Fcn2 : TransferFcn  Numerator=[10]  Denominator=[1 10]
  Out1 : Outport
  wires:
  Mux/1 -> Out1/1
  Transfer Fcn/1 -> Mux/1
  Transfer Fcn1/1 -> Mux/2
  Transfer Fcn2/1 -> Mux/3
  da_cmd/1 -> Transfer Fcn/1
  de_cmd/1 -> Transfer Fcn1/1
  dr_cmd/1 -> Transfer Fcn2/1

== system Fixed_Wing_Model/Visualization ==
  trans : Inport
  euler : Inport  Port=2
  Scope : Scope
  Simulation 3D Aircraft : aerolibsim3d/Simulation 3D Aircraft  Mesh=Sky Hogg  MeshPath=/MathWorksAerospaceContent/Vehicles/Aircraft/Custom/Mesh/SK_HL20.SK_HL20  MeshPathAT=/MathWorksAerospaceContent/Vehicles/Aircraft/AirTransport/Mesh/SK_AirTransport.SK_AirTransport  MeshPathGA=/MathWorksAerospaceContent/Vehicles/Aircraft/GeneralAviation/Mesh/SK_GeneralAviation.SK_GeneralAviation  AircraftColor=Red  ActorName=SimulinkVehicle1  Translation=[0 0 -2000; 0 0 0; 0 0 0; 0 0 0; 0 0 0; 0 0 0; 0 0 0; 0 0 0; 0 0 0; 0 0 0; 0 0 0]  Rotation=zeros( 11, 3 )  IsGHSensorEnabled=on  AreGHRaysVisible=off  IsOutputReshapeEnabled=off  GHRayLength=2500  GHBodyOffset=0.90  GHFrontTireRadius=0.21  GHLeftTireRadius=0.21  GHRightTireRadius=0.21  WoWSensorTolerance=0.05  LightsConfig=Automatic lights  LandingLightIntensity=300000  LandingLightConeAngle=15  CustomLeftLandingLightLocation=[0 0 0]  CustomLeftLandingLightOrientation=[0 0 0]  CustomRightLandingLightLocation=[0 0 0]  CustomRightLandingLightOrientation=[0 0 0]  TaxiLightIntensity=150000  TaxiLightConeAngle=36  CustomTaxiLightLocation=[0 0 0]  CustomTaxiLightOrientation=[0 0 0]  NavLightIntensity=500  PositionLightIntensity=500  StrobeLightIntensity=5000  WingtipStrobePeriod=1.5  WingtipStrobePulseWidth=6  TailStrobePeriod=1.5  TailStrobePulseWidth=6  BeaconLightIntensity=4000  BeaconPeriod=1.5  BeaconPulseWidth=10  SampleTime=-1  ActorType=SimulinkVehicle  ID=1  aMode=0  ActorTag=SimulinkVehicle1
  Simulation 3D Scene Configuration : sim3dlib/Simulation 3D Scene Configuration  Priority=0  ProjectFormat=Default Scenes  SceneDesc=Airport  ProjectName=C:\Program Files\MATLAB\R2023a\toolbox\shared\sim3d_projects\automotive_project\UE4\WindowsNoEditor\VehicleSimulation.exe  ScenePath=/Game/Maps/HwStrght  EnableOpenDRIVE=off  vehTagList={'Scene Origin';'SimulinkVehicle1'}  vehTag=SimulinkVehicle1  OpVisEn=off  Ts=1/100  EnableWindow=on  EnableRemoteAccess=off  EnableWeather=off  SunAltitude=40.0  SunAzimuth=90  clouds=10  wind=1  fog=0  rain=0  EnableGeospatial=off  OriginHeight=200  OriginLatitude=40.744652  OriginLongitude=-73.988864  MapStyle=Aerial  AdditionalAssetIDs=[]  UseAdvancedSunSky=off  SolarTime=11  TimeZone=-5  Day=21  Month=9  Year=2022  UseDaylightSavingTime=on  DSTStartDay=10  DSTStartMonth=3  DSTEndDay=3  DSTEndMonth=11  DSTSwitchHour=2  sensorTag=MainCamera1  sensorId=1  sensorName=MainCamera1  mountLoc=Origin  offsetFlag=off  tmountOffset=[0, 0, 0]  rmountOffset=[0, 0, 0]  HorizontalResolution=1280  VerticalResolution=720  HorizontalFOV=60  mountPoint=[0 0 0]  mountOrientation=[0 0 0]  aMode=0  ID=1  GeoTrigger=Inactive
  SkyHogg Rotation : Subsystem
  SkyHogg Translation : Subsystem
  Terminator : Terminator
  wires:
  Simulation 3D Aircraft/1 -> Scope/1
  Simulation 3D Aircraft/2 -> Terminator/1
  SkyHogg Rotation/1(Rotation) -> Simulation 3D Aircraft/2
  SkyHogg Translation/1(Translation) -> Simulation 3D Aircraft/1
  trans/1 -> SkyHogg Translation/1(trans)
  euler/1 -> SkyHogg Rotation/1(euler)

== system Fixed_Wing_Model/Wind_Model ==
  Aircraft_States : Inport
  Bus Creator : BusCreator  Inputs=2
  Bus Selector1 : BusSelector  OutputSignals=quat
  Constant{,1..5} (6 alike) : Constant  Value=0
  Mux : Mux  Inputs=3
  Mux1 : Mux  Inputs=3
  Quaternion Rotation : aerolibutil/Quaternion Rotation
  Wind_States : Outport
  wires:
  Constant2/1 -> Mux/3
  Constant1/1 -> Mux/2
  Constant/1 -> Mux/1
  [Aircraft_States] -> Bus Selector1/1
  Bus Selector1/1 -> Quaternion Rotation/1  "<quat>"
  Mux/1 -> Quaternion Rotation/2
  Quaternion Rotation/1 -> [Wind_Linear_Body]
  Constant3/1 -> Mux1/1
  Constant4/1 -> Mux1/2
  Constant5/1 -> Mux1/3
  Mux1/1 -> [Wind_Angular_Body]
  [Wind_Angular_Body] -> Bus Creator/2  "Wind_Angular_Body"
  [Wind_Linear_Body] -> Bus Creator/1  "Wind_Linear_Body"
  Bus Creator/1 -> Wind_States/1
  Aircraft_States/1 -> [Aircraft_States]

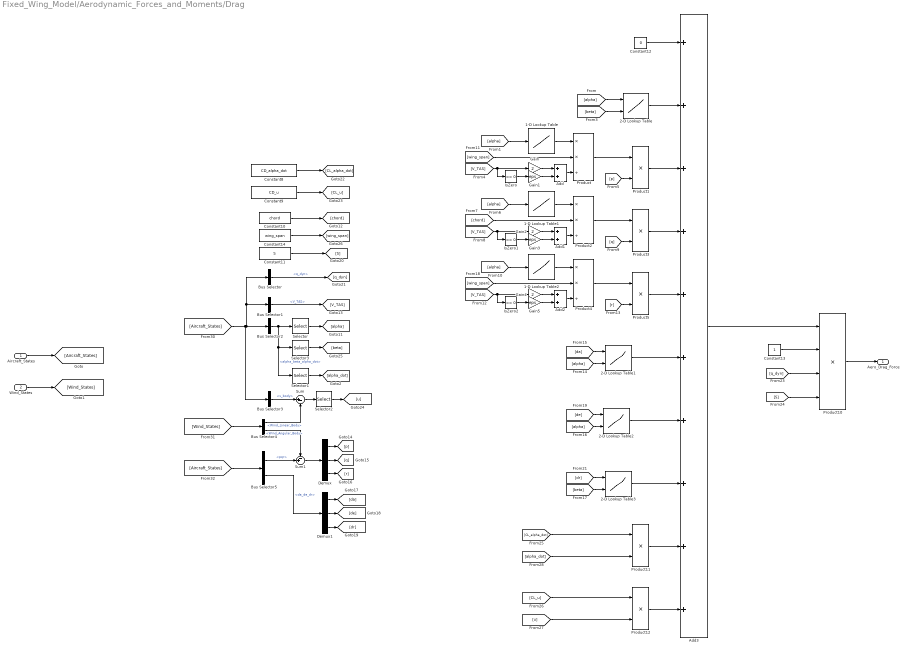
== system Fixed_Wing_Model/Aerodynamic_Forces_and_Moments/Drag ==
  Aircraft_States : Inport
  Wind_States : Inport  Port=2
  1-D Lookup Table : Lookup_n-D  NumberOfTableDimensions=1  BreakpointsForDimension1=Alpha  Table=CDp  InternalRulePriority=Speed  RndMeth=Simplest
  1-D Lookup Table1 : Lookup_n-D  NumberOfTableDimensions=1  BreakpointsForDimension1=Alpha  Table=CDq  InternalRulePriority=Speed  RndMeth=Simplest
  1-D Lookup Table2 : Lookup_n-D  NumberOfTableDimensions=1  BreakpointsForDimension1=Alpha  Table=CDr  InternalRulePriority=Speed  RndMeth=Simplest
  2-D Lookup Table : Lookup_n-D  BreakpointsForDimension1=Alpha  BreakpointsForDimension2=Beta  Table=CD_alpha_beta  InternalRulePriority=Speed  RndMeth=Simplest
      settings: InputPortMap=u0,u1
  2-D Lookup Table1 : Lookup_n-D  BreakpointsForDimension1=da  BreakpointsForDimension2=Alpha  Table=CDda  InternalRulePriority=Speed  RndMeth=Simplest
      settings: InputPortMap=u0,u1
  2-D Lookup Table2 : Lookup_n-D  BreakpointsForDimension1=da  BreakpointsForDimension2=Alpha  Table=CDde  InternalRulePriority=Speed  RndMeth=Simplest
      settings: InputPortMap=u0,u1
  2-D Lookup Table3 : Lookup_n-D  BreakpointsForDimension1=dr  BreakpointsForDimension2=Beta  Table=CDdr  InternalRulePriority=Speed  RndMeth=Simplest
      settings: InputPortMap=u0,u1
  Add : Sum
  Add1 : Sum
  Add2 : Sum
  Add3 : Sum  Inputs=10
  Bus Selector : BusSelector  OutputSignals=q_dyn
  Bus Selector1 : BusSelector  OutputSignals=V_TAS
  Bus Selector2 : BusSelector  OutputSignals=alpha_beta_alpha_dot
  Bus Selector3 : BusSelector  OutputSignals=v_body
  Bus Selector4 : BusSelector  OutputSignals=Wind_Linear_Body,Wind_Angular_Body
  Bus Selector5 : BusSelector  OutputSignals=pqr,da_de_dr
  Constant10 : Constant  Value=chord
  Constant11 : Constant  Value=S
  Constant12 : Constant  Value=0
  Constant13 : Constant
  Constant14 : Constant  Value=wing_span
  Constant8 : Constant  Value=CD_alpha_dot
  Constant9 : Constant  Value=CD_u
  Demux : Demux  Outputs=3
  Demux1 : Demux  Outputs=3
  Gain : Gain  Gain=2
  Gain1 : Gain  Gain=eps
  Gain2 : Gain  Gain=2
  Gain3 : Gain  Gain=eps
  Gain4 : Gain  Gain=2
  Gain5 : Gain  Gain=eps
  IsZero : simulink/Logic and Bit Operations/Compare To Zero  relop===  OutDataTypeStr=uint8
      settings: LibrarySourceBlock=|
      | simulink/Quick Insert/Logic and Bit
      | Operations/IsZero
  IsZero1 : simulink/Logic and Bit Operations/Compare To Zero  relop===  OutDataTypeStr=uint8
      settings: LibrarySourceBlock=|
      | simulink/Quick Insert/Logic and Bit
      | Operations/IsZero
  IsZero2 : simulink/Logic and Bit Operations/Compare To Zero  relop===  OutDataTypeStr=uint8
      settings: LibrarySourceBlock=|
      | simulink/Quick Insert/Logic and Bit
      | Operations/IsZero
  Product : Product  Inputs=**/
  Product{1,3,5,11..12} (5 alike) : Product
  Product10 : Product  Inputs=4
  Product2 : Product  Inputs=**/
  Product4 : Product  Inputs=**/
  Selector : Selector  InputPortWidth=3  IndexOptions=Index vector (dialog)  Indices=1  OutputSizes=1
  Selector1 : Selector  InputPortWidth=3  IndexOptions=Index vector (dialog)  Indices=3  OutputSizes=1
  Selector2 : Selector  InputPortWidth=3  IndexOptions=Index vector (dialog)  Indices=1  OutputSizes=1
  Selector3 : Selector  InputPortWidth=3  IndexOptions=Index vector (dialog)  Indices=2  OutputSizes=1
  Sum : Sum  Inputs=|+-
  Sum1 : Sum  Inputs=-+|
  Aero_Drag_Force : Outport  Unit=N*m
  wires:
  [u] -> Product12/2
  [alpha_dot] -> Product11/2
  [CL_u] -> Product12/1
  Product12/1 -> Add3/10
  [CL_alpha_dot] -> Product11/1
  Product11/1 -> Add3/9
  Constant11/1 -> [S]
  Constant9/1 -> [CL_u]
  Constant8/1 -> [CL_alpha_dot]
  Constant10/1 -> [chord]
  Product10/1 -> Aero_Drag_Force/1
  Demux/1 -> [p]
  Demux1/2 -> [de]
  Demux/2 -> [q]
  2-D Lookup Table3/1 -> Add3/8
  [de] -> 2-D Lookup Table2/1
  Product3/1 -> Add3/4
  [wing_span] -> Product4/2
  2-D Lookup Table/1 -> Add3/2
  IsZero/1 -> Gain1/1
  [p] -> Product1/2
  Product1/1 -> Add3/3
  Product/1 -> Product1/1
  [wing_span] -> Product/2
  [r] -> Product5/2
  IsZero1/1 -> Gain3/1
  [chord] -> Product2/2
  Demux1/1 -> [da]
  [q_dyn] -> Product10/3
  Gain2/1 -> Add1/1
  IsZero2/1 -> Gain5/1
  Gain3/1 -> Add1/2
  Gain4/1 -> Add2/1
  Gain/1 -> Add/1
  Product5/1 -> Add3/5
  [V_TAS] -> IsZero1/1, Gain2/1
  Demux/3 -> [r]
  Add3/1 -> Product10/1
  [q] -> Product3/2
  2-D Lookup Table1/1 -> Add3/6
  Product4/1 -> Product5/1
  Gain5/1 -> Add2/2
  Add1/1 -> Product2/3
  Constant13/1 -> Product10/2
  Product2/1 -> Product3/1
  Constant12/1 -> Add3/1
  Add/1 -> Product/3
  Add2/1 -> Product4/3
  [V_TAS] -> Gain/1, IsZero/1
  [V_TAS] -> Gain4/1, IsZero2/1
  Gain1/1 -> Add/2
  [S] -> Product10/4
  2-D Lookup Table2/1 -> Add3/7
  Demux1/3 -> [dr]
  Aircraft_States/1 -> [Aircraft_States]
  Wind_States/1 -> [Wind_States]
  [Aircraft_States] -> Bus Selector3/1, Bus Selector/1, Bus Selector1/1, Bus Selector2/1
  Bus Selector/1 -> [q_dyn]  "<q_dyn>"
  Bus Selector1/1 -> [V_TAS]  "<V_TAS>"
  Bus Selector2/1 -> Selector3/1, Selector1/1, Selector/1  "<alpha_beta_alpha_dot>"
  Selector/1 -> [alpha]
  Selector1/1 -> [alpha_dot]
  Selector2/1 -> [u]
  [Wind_States] -> Bus Selector4/1
  Bus Selector4/1 -> Sum/2  "<Wind_Linear_Body>"
  Bus Selector3/1 -> Sum/1  "<v_body>"
  Sum/1 -> Selector2/1
  Sum1/1 -> Demux/1
  Bus Selector4/2 -> Sum1/1  "<Wind_Angular_Body>"
  [Aircraft_States] -> Bus Selector5/1
  Bus Selector5/1 -> Sum1/2  "<pqr>"
  Bus Selector5/2 -> Demux1/1  "<da_de_dr>"
  Selector3/1 -> [beta]
  [alpha] -> 2-D Lookup Table/1
  [beta] -> 2-D Lookup Table/2
  1-D Lookup Table/1 -> Product/1
  [alpha] -> 1-D Lookup Table/1
  1-D Lookup Table1/1 -> Product2/1
  [alpha] -> 1-D Lookup Table1/1
  1-D Lookup Table2/1 -> Product4/1
  [alpha] -> 1-D Lookup Table2/1
  [alpha] -> 2-D Lookup Table1/2
  [da] -> 2-D Lookup Table1/1
  [alpha] -> 2-D Lookup Table2/2
  [dr] -> 2-D Lookup Table3/1
  [beta] -> 2-D Lookup Table3/2
  Constant14/1 -> [wing_span]

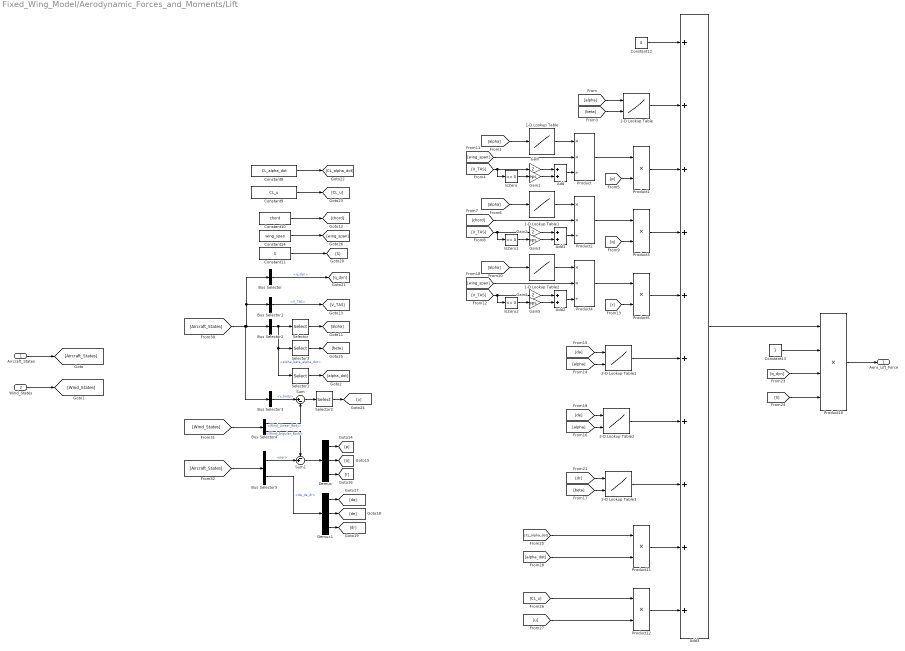
== system Fixed_Wing_Model/Aerodynamic_Forces_and_Moments/Lift ==
  Aircraft_States : Inport
  Wind_States : Inport  Port=2
  1-D Lookup Table : Lookup_n-D  NumberOfTableDimensions=1  BreakpointsForDimension1=Alpha  Table=CLp  InternalRulePriority=Speed  RndMeth=Simplest
  1-D Lookup Table1 : Lookup_n-D  NumberOfTableDimensions=1  BreakpointsForDimension1=Alpha  Table=CLq  InternalRulePriority=Speed  RndMeth=Simplest
  1-D Lookup Table2 : Lookup_n-D  NumberOfTableDimensions=1  BreakpointsForDimension1=Alpha  Table=CLr  InternalRulePriority=Speed  RndMeth=Simplest
  2-D Lookup Table : Lookup_n-D  BreakpointsForDimension1=Alpha  BreakpointsForDimension2=Beta  Table=CL_alpha_beta  InternalRulePriority=Speed  RndMeth=Simplest
      settings: InputPortMap=u0,u1
  2-D Lookup Table1 : Lookup_n-D  BreakpointsForDimension1=da  BreakpointsForDimension2=Alpha  Table=CLda  InternalRulePriority=Speed  RndMeth=Simplest
      settings: InputPortMap=u0,u1
  2-D Lookup Table2 : Lookup_n-D  BreakpointsForDimension1=da  BreakpointsForDimension2=Alpha  Table=CLde  InternalRulePriority=Speed  RndMeth=Simplest
      settings: InputPortMap=u0,u1
  2-D Lookup Table3 : Lookup_n-D  BreakpointsForDimension1=dr  BreakpointsForDimension2=Beta  Table=CLdr  InternalRulePriority=Speed  RndMeth=Simplest
      settings: InputPortMap=u0,u1
  Add : Sum
  Add1 : Sum
  Add2 : Sum
  Add3 : Sum  Inputs=10
  Bus Selector : BusSelector  OutputSignals=q_dyn
  Bus Selector1 : BusSelector  OutputSignals=V_TAS
  Bus Selector2 : BusSelector  OutputSignals=alpha_beta_alpha_dot
  Bus Selector3 : BusSelector  OutputSignals=v_body
  Bus Selector4 : BusSelector  OutputSignals=Wind_Linear_Body,Wind_Angular_Body
  Bus Selector5 : BusSelector  OutputSignals=pqr,da_de_dr
  Constant10 : Constant  Value=chord
  Constant11 : Constant  Value=S
  Constant12 : Constant  Value=0
  Constant13 : Constant
  Constant14 : Constant  Value=wing_span
  Constant8 : Constant  Value=CL_alpha_dot
  Constant9 : Constant  Value=CL_u
  Demux : Demux  Outputs=3
  Demux1 : Demux  Outputs=3
  Gain : Gain  Gain=2
  Gain1 : Gain  Gain=eps
  Gain2 : Gain  Gain=2
  Gain3 : Gain  Gain=eps
  Gain4 : Gain  Gain=2
  Gain5 : Gain  Gain=eps
  IsZero : simulink/Logic and Bit Operations/Compare To Zero  relop===  OutDataTypeStr=uint8
      settings: LibrarySourceBlock=|
      | simulink/Quick Insert/Logic and Bit
      | Operations/IsZero
  IsZero1 : simulink/Logic and Bit Operations/Compare To Zero  relop===  OutDataTypeStr=uint8
      settings: LibrarySourceBlock=|
      | simulink/Quick Insert/Logic and Bit
      | Operations/IsZero
  IsZero2 : simulink/Logic and Bit Operations/Compare To Zero  relop===  OutDataTypeStr=uint8
      settings: LibrarySourceBlock=|
      | simulink/Quick Insert/Logic and Bit
      | Operations/IsZero
  Product : Product  Inputs=**/
  Product{1,3,5,11..12} (5 alike) : Product
  Product10 : Product  Inputs=4
  Product2 : Product  Inputs=**/
  Product4 : Product  Inputs=**/
  Selector : Selector  InputPortWidth=3  IndexOptions=Index vector (dialog)  Indices=1  OutputSizes=1
  Selector1 : Selector  InputPortWidth=3  IndexOptions=Index vector (dialog)  Indices=3  OutputSizes=1
  Selector2 : Selector  InputPortWidth=3  IndexOptions=Index vector (dialog)  Indices=1  OutputSizes=1
  Selector3 : Selector  InputPortWidth=3  IndexOptions=Index vector (dialog)  Indices=2  OutputSizes=1
  Sum : Sum  Inputs=|+-
  Sum1 : Sum  Inputs=-+|
  Aero_Lift_Force : Outport  Unit=N*m
  wires:
  [u] -> Product12/2
  [alpha_dot] -> Product11/2
  [CL_u] -> Product12/1
  Product12/1 -> Add3/10
  [CL_alpha_dot] -> Product11/1
  Product11/1 -> Add3/9
  Constant11/1 -> [S]
  Constant9/1 -> [CL_u]
  Constant8/1 -> [CL_alpha_dot]
  Constant10/1 -> [chord]
  Product10/1 -> Aero_Lift_Force/1
  Demux/1 -> [p]
  Demux1/2 -> [de]
  Demux/2 -> [q]
  2-D Lookup Table3/1 -> Add3/8
  [de] -> 2-D Lookup Table2/1
  Product3/1 -> Add3/4
  [wing_span] -> Product4/2
  2-D Lookup Table/1 -> Add3/2
  IsZero/1 -> Gain1/1
  [p] -> Product1/2
  Product1/1 -> Add3/3
  Product/1 -> Product1/1
  [wing_span] -> Product/2
  [r] -> Product5/2
  IsZero1/1 -> Gain3/1
  [chord] -> Product2/2
  Demux1/1 -> [da]
  [q_dyn] -> Product10/3
  Gain2/1 -> Add1/1
  IsZero2/1 -> Gain5/1
  Gain3/1 -> Add1/2
  Gain4/1 -> Add2/1
  Gain/1 -> Add/1
  Product5/1 -> Add3/5
  [V_TAS] -> IsZero1/1, Gain2/1
  Demux/3 -> [r]
  Add3/1 -> Product10/1
  [q] -> Product3/2
  2-D Lookup Table1/1 -> Add3/6
  Product4/1 -> Product5/1
  Gain5/1 -> Add2/2
  Add1/1 -> Product2/3
  Constant13/1 -> Product10/2
  Product2/1 -> Product3/1
  Constant12/1 -> Add3/1
  Add/1 -> Product/3
  Add2/1 -> Product4/3
  [V_TAS] -> Gain/1, IsZero/1
  [V_TAS] -> Gain4/1, IsZero2/1
  Gain1/1 -> Add/2
  [S] -> Product10/4
  2-D Lookup Table2/1 -> Add3/7
  Demux1/3 -> [dr]
  Aircraft_States/1 -> [Aircraft_States]
  Wind_States/1 -> [Wind_States]
  [Aircraft_States] -> Bus Selector3/1, Bus Selector/1, Bus Selector1/1, Bus Selector2/1
  Bus Selector/1 -> [q_dyn]  "<q_dyn>"
  Bus Selector1/1 -> [V_TAS]  "<V_TAS>"
  Bus Selector2/1 -> Selector3/1, Selector1/1, Selector/1  "<alpha_beta_alpha_dot>"
  Selector/1 -> [alpha]
  Selector1/1 -> [alpha_dot]
  Selector2/1 -> [u]
  [Wind_States] -> Bus Selector4/1
  Bus Selector4/1 -> Sum/2  "<Wind_Linear_Body>"
  Bus Selector3/1 -> Sum/1  "<v_body>"
  Sum/1 -> Selector2/1
  Sum1/1 -> Demux/1
  Bus Selector4/2 -> Sum1/1  "<Wind_Angular_Body>"
  [Aircraft_States] -> Bus Selector5/1
  Bus Selector5/1 -> Sum1/2  "<pqr>"
  Bus Selector5/2 -> Demux1/1  "<da_de_dr>"
  Selector3/1 -> [beta]
  [alpha] -> 2-D Lookup Table/1
  [beta] -> 2-D Lookup Table/2
  1-D Lookup Table/1 -> Product/1
  [alpha] -> 1-D Lookup Table/1
  1-D Lookup Table1/1 -> Product2/1
  [alpha] -> 1-D Lookup Table1/1
  1-D Lookup Table2/1 -> Product4/1
  [alpha] -> 1-D Lookup Table2/1
  [alpha] -> 2-D Lookup Table1/2
  [da] -> 2-D Lookup Table1/1
  [alpha] -> 2-D Lookup Table2/2
  [dr] -> 2-D Lookup Table3/1
  [beta] -> 2-D Lookup Table3/2
  Constant14/1 -> [wing_span]
